simulink model "solucion_1_block"  (R2020b)
settings: Solver=VariableStepAuto  StartTime=0.0  StopTime=10  RelTol=1e-3
model workspace (MAT data in the model file):
  Symbol_period = 2e-06
  alpha_fll = 0.392699081699
  gamma_fll = 0.001
  gamma_pll = 0.01
  phase_offset = 0
  ro_fll = 0.001
  ro_pll = 0.01
values from neighbouring files (symbols this model uses):
  doppler = [t', d']    [generate_doppler.m]
undefined symbols (not defined in the file or in its folder): j
libraries: commdigbbndpm3 x5, commutil2 x2, commsink2 x2, commchan3 x1, simulink x1, commrandsrc3 x1
settings Model: OrderedModelArguments=off  Creator=Raul  LastModifiedBy=Raul
settings DataIOCC: ReturnWorkspaceOutputs=off

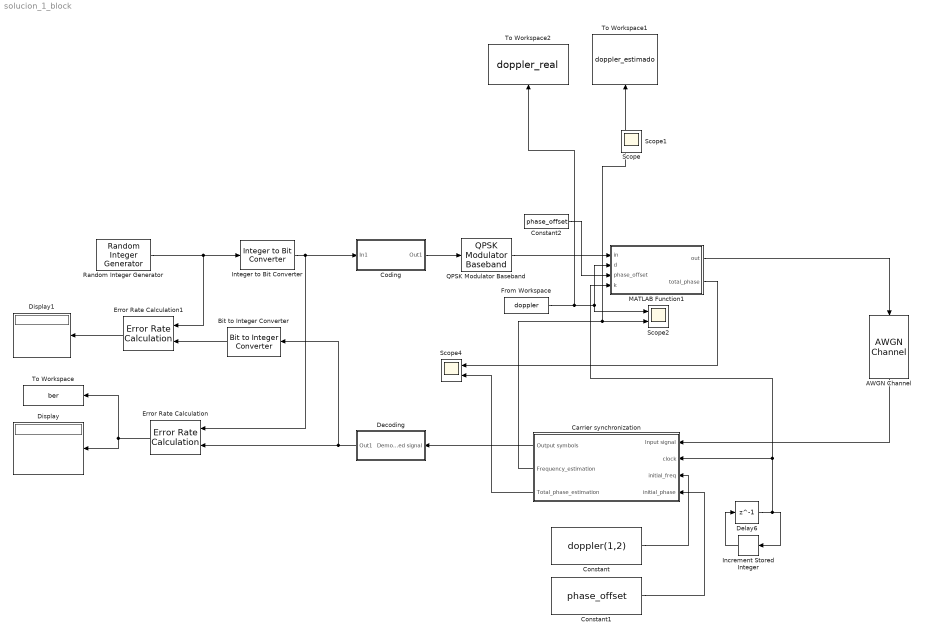
== system solucion_1_block ==
  AWGN Channel : commchan3/AWGN Channel  InputProcessing=Columns as channels (frame based)  seed=57  noiseMode="Signal to noise ratio  (Eb/No)"  EbNodB=8  EsNodB=10  SNRdB=10  bitsPerSym=2  Ps=1  Tsym=Symbol_period  variance=1
  Bit to Integer Converter : commutil2/Bit to Integer Converter  nbits=2  bitOrder=MSB first  signedOutputValues=Unsigned  outDtype=Inherit via internal rule  outDtypeSigned=Inherit via internal rule
  Carrier synchronization : Subsystem
  Coding : Subsystem
  Constant : Constant  Value=doppler(1,2)
  Constant1 : Constant  Value=phase_offset
  Constant2 : Constant  Value=phase_offset  SampleTime=Symbol_period
  Decoding : Subsystem
  Delay6 : Delay  DelayLength=1  InitialCondition=0
  Display : Display
      settings: Format=short_e
  Display1 : Display
      settings: Format=short_e
  Error Rate Calculation : commsink2/Error Rate Calculation  N=0  st_delay=0  cp_mode=Entire frame  subframe=[]  PMode=Port  WsName=ErrorVec  RsMode2=off  stop=off  numErr=100  maxBits=1e6
  Error Rate Calculation1 : commsink2/Error Rate Calculation  N=0  st_delay=0  cp_mode=Entire frame  subframe=[]  PMode=Port  WsName=ErrorVec  RsMode2=off  stop=off  numErr=100  maxBits=1e6
  From Workspace : FromWorkspace  VariableName=doppler  SampleTime=-1  OutputAfterFinalValue=Holding final value
  Increment Stored Integer : simulink/Additional Math & Discrete/Additional Math: Increment - Decrement/Increment Stored Integer
  Integer to Bit Converter : commutil2/Integer to Bit Converter  nbits=2  signedInputValues=Unsigned  bitOrder=MSB first  outDtype=Inherit via internal rule
  MATLAB Function1 : MATLAB Function  TreatAsAtomicUnit=on
  QPSK Modulator Baseband : commdigbbndpm3/QPSK Modulator Baseband  InType=Bit  Enc=Gray  Ph=pi/4  outDtype=double  outWordLen=16  outUDDataType=sfix(16)  outFracLenMode=Best precision  outFracLen=15  outDataTypeStr=double  outLastDataTypeStr=double
  Random Integer Generator : commrandsrc3/Random Integer Generator  SetSize=4  SeedSource=Parameter  Seed=456  SampleTime=Symbol_period  SamplesPerFrame=1  OutputDataType=uint8  SimulateUsing=Interpreted execution
  Scope2 : Scope  NumInputPorts=2
  Scope4 : Scope  NumInputPorts=2
  To Workspace : ToWorkspace  VariableName=ber  SampleTime=-1
      settings: MaxDataPoints=1  Save2DSignal=2-D array (concatenate along first dimension)
  To Workspace1 : ToWorkspace  VariableName=doppler_estimado  SampleTime=-1
      settings: Save2DSignal=2-D array (concatenate along first dimension)
  To Workspace2 : ToWorkspace  VariableName=doppler_real  SampleTime=-1
      settings: Save2DSignal=2-D array (concatenate along first dimension)
  Scope : Scope
  Scope1 : Scope
  wires:
  Random Integer Generator/1 -> Error Rate Calculation1/1, Integer to Bit Converter/1
  Bit to Integer Converter/1 -> Error Rate Calculation1/2
  Integer to Bit Converter/1 -> Error Rate Calculation/1, Coding/1(In1)
  Error Rate Calculation/1 -> Display/1, To Workspace/1
  Error Rate Calculation1/1 -> Display1/1
  Coding/1(Out1) -> QPSK Modulator Baseband/1
  Decoding/1(Out1) -> Error Rate Calculation/2, Bit to Integer Converter/1
  Delay6/1 -> MATLAB Function1/4(k), Carrier synchronization/2(clock), Increment Stored Integer/1
  Increment Stored Integer/1 -> Delay6/1
  MATLAB Function1/1(out) -> AWGN Channel/1
  QPSK Modulator Baseband/1 -> MATLAB Function1/1(in)
  From Workspace/1 -> To Workspace2/1, MATLAB Function1/2(d), Scope2/1
  Constant2/1 -> MATLAB Function1/3(phase_offset)
  AWGN Channel/1 -> Carrier synchronization/1(Input signal)
  Carrier synchronization/1(Output symbols) -> Decoding/1(Demodulated signal)
  Constant/1 -> Carrier synchronization/3(initial_freq)
  Carrier synchronization/2(Frequency_estimation) -> Scope2/2, To Workspace1/1
  MATLAB Function1/2(total_phase) -> Scope4/1
  Carrier synchronization/3(Total_phase_estimation) -> Scope4/2
  Constant1/1 -> Carrier synchronization/4(initial_phase)

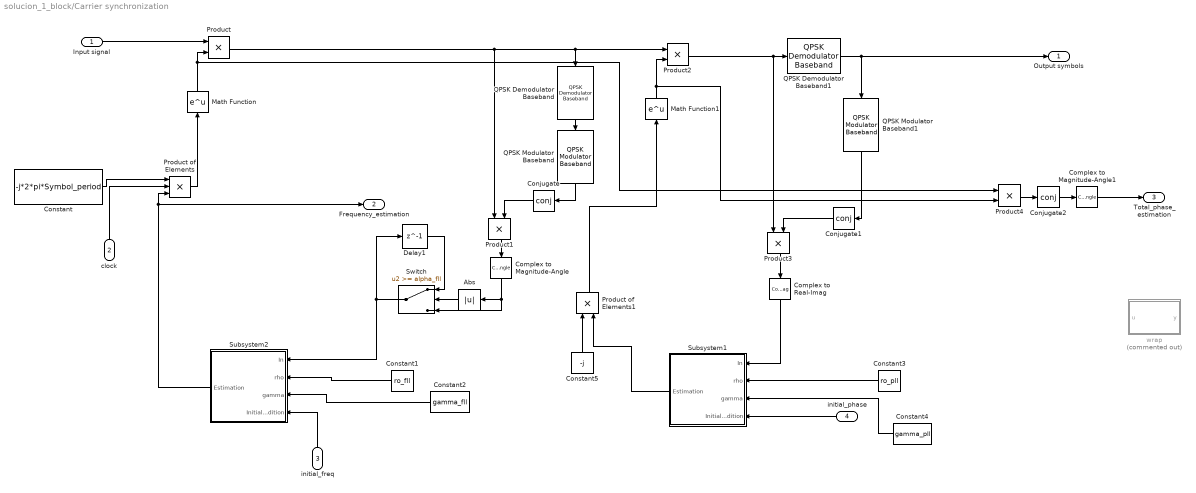
== system solucion_1_block/Carrier synchronization ==
  Input signal : Inport
  clock : Inport  Port=2
  initial_freq : Inport  Port=3
  initial_phase : Inport  Port=4
  Abs : Abs
  Complex to Magnitude-Angle : ComplexToMagnitudeAngle  Output=Angle
  Complex to Magnitude-Angle1 : ComplexToMagnitudeAngle  Output=Angle
  Complex to Real-Imag : ComplexToRealImag  Output=Imag
  Conjugate : Math  Operator=conj  SignedPower=on  RndMeth=Zero  SaturateOnIntegerOverflow=on
  Conjugate1 : Math  Operator=conj  SignedPower=on  RndMeth=Zero  SaturateOnIntegerOverflow=on
  Conjugate2 : Math  Operator=conj  SignedPower=on  RndMeth=Zero  SaturateOnIntegerOverflow=on
  Constant : Constant  Value=-j*2*pi*Symbol_period
  Constant1 : Constant  Value=ro_fll
  Constant2 : Constant  Value=gamma_fll
  Constant3 : Constant  Value=ro_pll
  Constant4 : Constant  Value=gamma_pll
  Constant5 : Constant  Value=-j
  Delay1 : Delay  DelayLength=1  InitialCondition=0
  Math Function : Math  SaturateOnIntegerOverflow=on
  Math Function1 : Math  SaturateOnIntegerOverflow=on
  Product{,1..4} (5 alike) : Product
  Product of Elements : Product  Inputs=***
  Product of Elements1 : Product  Inputs=**
  QPSK Demodulator Baseband : commdigbbndpm3/QPSK Demodulator Baseband  OutType=Integer  DecType=Hard decision  VarSource=Dialog  Variance=1  Dec=Gray  Ph=pi/4  outDtype1=Inherit via internal rule  outDtype2=Inherit via internal rule  derotateFactorWordLen=16  derotateFactorDataTypeStr=Inherit: Same word length as input  derotateFactorLastDataTypeStr=Inherit: Same word length as input
  QPSK Demodulator Baseband1 : commdigbbndpm3/QPSK Demodulator Baseband  OutType=Bit  DecType=Hard decision  VarSource=Dialog  Variance=1  Dec=Gray  Ph=pi/4  outDtype1=Inherit via internal rule  outDtype2=Inherit via internal rule  derotateFactorWordLen=16  derotateFactorDataTypeStr=Inherit: Same word length as input  derotateFactorLastDataTypeStr=Inherit: Same word length as input
  QPSK Modulator Baseband : commdigbbndpm3/QPSK Modulator Baseband  InType=Integer  Enc=Gray  Ph=pi/4  outDtype=double  outWordLen=16  outUDDataType=sfix(16)  outFracLenMode=Best precision  outFracLen=15  outDataTypeStr=double  outLastDataTypeStr=double
  QPSK Modulator Baseband1 : commdigbbndpm3/QPSK Modulator Baseband  InType=Bit  Enc=Gray  Ph=pi/4  outDtype=double  outWordLen=16  outUDDataType=sfix(16)  outFracLenMode=Best precision  outFracLen=15  outDataTypeStr=double  outLastDataTypeStr=double
  Subsystem1 : Subsystem
  Subsystem2 : Subsystem
  Switch : Switch  Threshold=alpha_fll  OutDataTypeStr=double
  wrap : MATLAB Function  Commented=on  TreatAsAtomicUnit=on
  Output symbols : Outport
  Frequency_estimation : Outport  Port=2
  Total_phase_estimation : Outport  Port=3
  wires:
  Input signal/1 -> Product/1
  Constant/1 -> Product of Elements/1
  clock/1 -> Product of Elements/2
  Product of Elements/1 -> Math Function/1
  Math Function/1 -> Product4/1, Product/2
  Constant1/1 -> Subsystem2/2(rho)
  Constant2/1 -> Subsystem2/3(gamma)
  Switch/1 -> Delay1/1, Subsystem2/1(In)
  Product/1 -> Product2/1, QPSK Demodulator Baseband/1, Product1/1
  QPSK Demodulator Baseband/1 -> QPSK Modulator Baseband/1
  QPSK Modulator Baseband/1 -> Conjugate/1
  Conjugate/1 -> Product1/2
  Abs/1 -> Switch/2
  Delay1/1 -> Switch/1
  Math Function1/1 -> Product2/2, Product4/2
  Product2/1 -> Product3/1, QPSK Demodulator Baseband1/1
  Conjugate1/1 -> Product3/2
  QPSK Demodulator Baseband1/1 -> Output symbols/1, QPSK Modulator Baseband1/1
  QPSK Modulator Baseband1/1 -> Conjugate1/1
  Product3/1 -> Complex to Real-Imag/1
  Constant4/1 -> Subsystem1/3(gamma)
  Constant5/1 -> Product of Elements1/1
  Product of Elements1/1 -> Math Function1/1
  Product1/1 -> Complex to Magnitude-Angle/1
  Complex to Magnitude-Angle/1 -> Switch/3, Abs/1
  Product4/1 -> Conjugate2/1
  Conjugate2/1 -> Complex to Magnitude-Angle1/1
  Complex to Magnitude-Angle1/1 -> Total_phase_estimation/1
  initial_phase/1 -> Subsystem1/4(Initial_condition)
  initial_freq/1 -> Subsystem2/4(Initial_condition)
  Subsystem2/1(Estimation) -> Frequency_estimation/1, Product of Elements/3
  Subsystem1/1(Estimation) -> Product of Elements1/2
  Complex to Real-Imag/1 -> Subsystem1/1(In)
  Constant3/1 -> Subsystem1/2(rho)

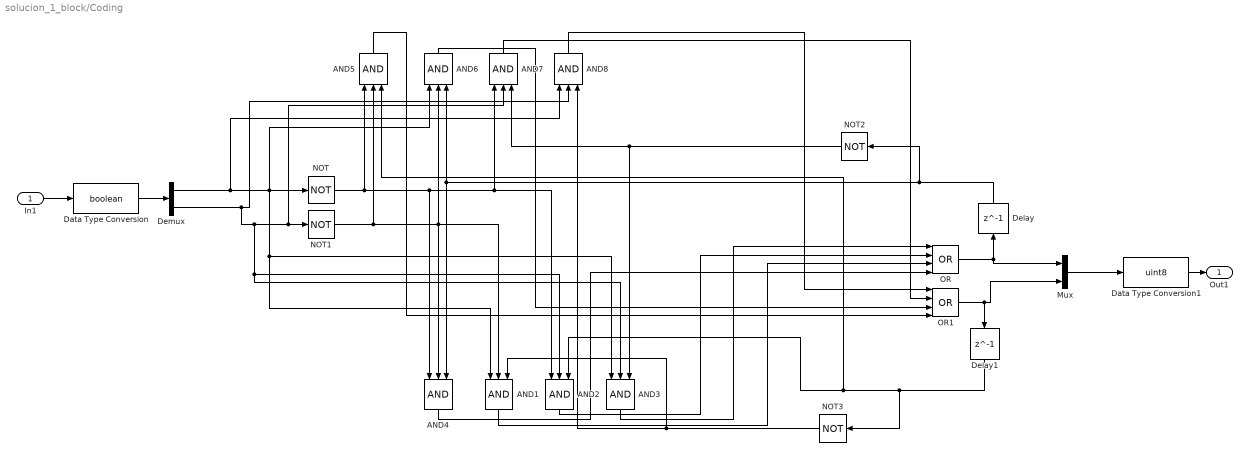
== system solucion_1_block/Coding ==
  In1 : Inport
  AND{1..8} (8 alike) : Logic  Inputs=3  IconShape=distinctive  AllPortsSameDT=off  OutDataTypeStr=boolean
  Data Type Conversion : DataTypeConversion  OutDataTypeStr=boolean
  Data Type Conversion1 : DataTypeConversion  OutDataTypeStr=uint8
  Delay : Delay  DelayLength=1  InitialCondition=0
  Delay1 : Delay  DelayLength=1  InitialCondition=0
  Demux : Demux  Outputs=2
  Mux : Mux  Inputs=2
  NOT{,1..3} (4 alike) : Logic  Operator=NOT  IconShape=distinctive  AllPortsSameDT=off  OutDataTypeStr=boolean
  OR : Logic  Operator=OR  Inputs=4  IconShape=distinctive  AllPortsSameDT=off  OutDataTypeStr=boolean
  OR1 : Logic  Operator=OR  Inputs=4  IconShape=distinctive  AllPortsSameDT=off  OutDataTypeStr=boolean
  Out1 : Outport
  wires:
  Demux/1 -> AND8/1, AND6/1, AND3/1, AND1/1, NOT/1
  OR/1 -> Delay/1, Mux/1
  OR1/1 -> Mux/2, Delay1/1
  Delay/1 -> AND6/3, AND4/3, NOT2/1
  Demux/2 -> AND8/2, AND2/2, AND3/2, AND7/2, NOT1/1
  Delay1/1 -> NOT3/1, AND5/3, AND2/3
  NOT/1 -> AND7/1, AND2/1, AND4/1, AND5/1
  NOT1/1 -> AND6/2, AND1/2, AND4/2, AND5/2
  Mux/1 -> Data Type Conversion1/1
  NOT3/1 -> AND8/3, AND1/3
  NOT2/1 -> AND7/3, AND3/3
  AND3/1 -> OR/1
  AND2/1 -> OR/2
  AND1/1 -> OR/3
  AND4/1 -> OR/4
  AND8/1 -> OR1/1
  AND6/1 -> OR1/3
  AND7/1 -> OR1/2
  AND5/1 -> OR1/4
  Data Type Conversion/1 -> Demux/1
  In1/1 -> Data Type Conversion/1
  Data Type Conversion1/1 -> Out1/1

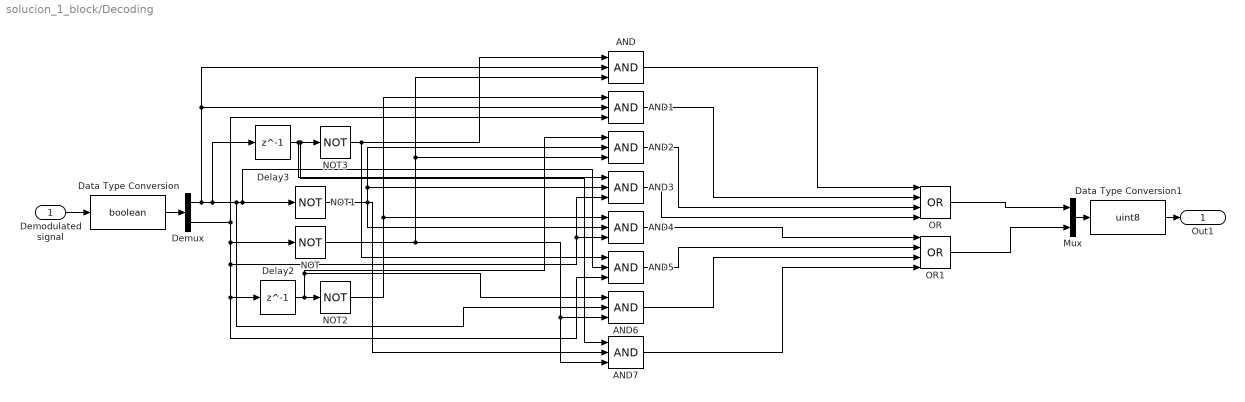
== system solucion_1_block/Decoding ==
  Demodulated signal : Inport
  AND{,1..7} (8 alike) : Logic  Inputs=3  IconShape=distinctive  AllPortsSameDT=off  OutDataTypeStr=boolean
  Data Type Conversion : DataTypeConversion  OutDataTypeStr=boolean
  Data Type Conversion1 : DataTypeConversion  OutDataTypeStr=uint8
  Delay2 : Delay  DelayLength=1  InitialCondition=0
  Delay3 : Delay  DelayLength=1  InitialCondition=0
  Demux : Demux  Outputs=2
  Mux : Mux  Inputs=2
  NOT{,1..3} (4 alike) : Logic  Operator=NOT  IconShape=distinctive  AllPortsSameDT=off  OutDataTypeStr=boolean
  OR : Logic  Operator=OR  Inputs=4  IconShape=distinctive  AllPortsSameDT=off  OutDataTypeStr=boolean
  OR1 : Logic  Operator=OR  Inputs=4  IconShape=distinctive  AllPortsSameDT=off  OutDataTypeStr=boolean
  Out1 : Outport
  wires:
  OR/1 -> Mux/1
  Demux/2 -> AND4/3, AND3/3, AND5/3, Delay2/1, NOT/1, AND1/3
  Delay2/1 -> AND6/1, AND2/1, NOT2/1
  Demux/1 -> AND1/2, AND/2, Delay3/1, AND6/2, AND5/2, NOT1/1
  Delay3/1 -> AND3/1, AND7/1, NOT3/1
  AND7/1 -> OR1/4
  AND6/1 -> OR1/3
  AND5/1 -> OR1/2
  AND4/1 -> OR1/1
  AND/1 -> OR/1
  AND1/1 -> OR/2
  AND2/1 -> OR/3
  AND3/1 -> OR/4
  OR1/1 -> Mux/2
  NOT3/1 -> AND5/1, AND/1
  NOT/1 -> AND7/3, AND6/3, AND2/3, AND/3
  NOT2/1 -> AND4/1, AND1/1
  NOT1/1 -> AND7/2, AND3/2, AND2/2, AND4/2
  Demodulated signal/1 -> Data Type Conversion/1
  Data Type Conversion/1 -> Demux/1
  Mux/1 -> Data Type Conversion1/1
  Data Type Conversion1/1 -> Out1/1

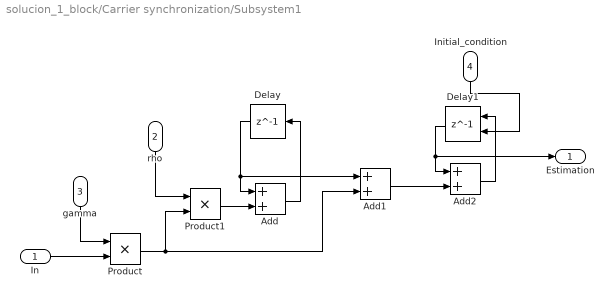
== system solucion_1_block/Carrier synchronization/Subsystem1 ==
  In : Inport
  rho : Inport  Port=2
  gamma : Inport  Port=3
  Initial_condition : Inport  Port=4
  Add : Sum
  Add1 : Sum
  Add2 : Sum
  Delay : Delay  DelayLength=1  InitialCondition=0
  Delay1 : Delay  DelayLength=1  InitialConditionSource=Input port  InitialCondition=0
      settings: InputPortMap=u0,p4
  Product : Product
  Product1 : Product
  Estimation : Outport
  wires:
  In/1 -> Product/2
  gamma/1 -> Product/1
  Product/1 -> Product1/2, Add1/2
  rho/1 -> Product1/1
  Add/1 -> Delay/1
  Product1/1 -> Add/2
  Delay/1 -> Add1/1, Add/1
  Add1/1 -> Add2/2
  Add2/1 -> Delay1/1
  Delay1/1 -> Estimation/1, Add2/1
  Initial_condition/1 -> Delay1/2

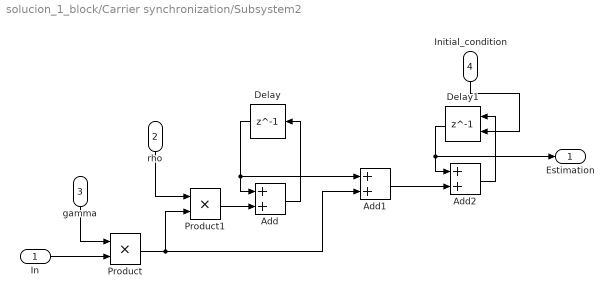
== system solucion_1_block/Carrier synchronization/Subsystem2 ==
  In : Inport
  rho : Inport  Port=2
  gamma : Inport  Port=3
  Initial_condition : Inport  Port=4
  Add : Sum
  Add1 : Sum
  Add2 : Sum
  Delay : Delay  DelayLength=1  InitialCondition=0
  Delay1 : Delay  DelayLength=1  InitialConditionSource=Input port  InitialCondition=0
      settings: InputPortMap=u0,p4
  Product : Product
  Product1 : Product
  Estimation : Outport
  wires:
  In/1 -> Product/2
  gamma/1 -> Product/1
  Product/1 -> Product1/2, Add1/2
  rho/1 -> Product1/1
  Add/1 -> Delay/1
  Product1/1 -> Add/2
  Delay/1 -> Add1/1, Add/1
  Add1/1 -> Add2/2
  Add2/1 -> Delay1/1
  Delay1/1 -> Estimation/1, Add2/1
  Initial_condition/1 -> Delay1/2

== matlab function solucion_1_block/MATLAB Function1 ==
  data: in input; d input; out output; phase_offset input; k input; total_phase output
function [out,total_phase] = apply_doppler_and_phase(in, d,phase_offset,k)
    T = 2e-6;
    factor = exp(1j*((2*pi*d.*k*T)+phase_offset));
    out = in * factor;
    total_phase = angle(factor);
end

== matlab function solucion_1_block/Carrier synchronization/wrap ==
  data: u input; y output
function y = wrap_phase(u)
    y = wrapToPi(u);
end
